simulink model "ColdGas_GNC_Model"  (R2024a)
settings: Solver=VariableStepAuto  StartTime=0.0  StopTime=tFinal  RelTol=1e-3
values from neighbouring files (symbols this model uses):
  Aero_Forces_On = 1    [run_Lander_GNC_Sim.m]
  Cd = 1.2    [Load_Aero_Data.m]
  CE_Direction = [0 0 -1]    [Load_VehicleParams.m]
  CE_ISP = 40    [Load_VehicleParams.m]
  CE_Location = [0 0 0]    [Load_VehicleParams.m]
  CE_tau = 0.100    (= 0.1)    [Load_VehicleParams.m]
  CE_tDelay = 0.030    (= 0.03)    [Load_VehicleParams.m]
  CE_Thrust = 132    [Load_VehicleParams.m]
  Cm_Lookup = [Phi'  Cm]    [Load_Aero_Data.m]
  Fan_den = [1  70.7  2500]    [Load_VehicleParams.m]
  Fan_num = 2500    [Load_VehicleParams.m]
  fan_thrust_Poly = [0.0009987  -0.04316  4.44]    [Load_VehicleParams.m]
  FlightPlan_Lateral = [0 1 5 9 13 17 20 30 30.1 30.2 2 2 ... (40 elements, 10x4)]    [Lateral_Flight_Schedule_10m.mat]    (also in Lateral_Flight_Schedule_14.mat = [0 1 11 12 13 22 29.4 29.6 29.8 30 2 2 ... (40 elements, 10x; Lateral_Flight_Schedule_15m.mat = [0 1 8.5 9 13 17 20 30 30.1 30.2 2 2 ... (40 elements, 10x4); Lateral_Flight_Schedule_2.mat = [0 3 4 6 13 17 20 30 30.1 30.2 2 2 ... (40 elements, 10x4)]; Lateral_Flight_Schedule_22.mat = [0 3 3.2 3.5 15 20 30 30.1 30.2 30.3 2 2 ... (40 elements, 1)
  FlightPlan_Vertical = [0 3 3.2 13 30 30.1 30.2 30.3 30.4 30.5 1 1 ... (30 elements, 10x3)]    [Vertical_Flight_Schedule_10m.mat]    (also in Vertical_Flight_Schedule_14.mat = [0 3 3.01 17 29 29.2 29.4 29.6 29.8 30 1 1 ... (30 elements,; Vertical_Flight_Schedule_3_15_20.mat = [0 3 3.01 15 20 29.2 29.4 29.6 29.8 30 1 1 ... (30 elements,; Vertical_Flight_Schedule_3ms.mat = [0 3 3.2 16 30 30.1 30.2 30.3 30.4 30.5 1 1 ... (30 elements)
  g = 9.807    [Load_VehicleParams.m]
  gustDuration = 9    [Load_Aero_Data.m]
  gustFactor = 1.0    (= 1)    [Load_Aero_Data.m]
  hFinal = 0.28    [run_Lander_GNC_Sim.m]
  I = [ 12  0  0 ... (first row only)    [Load_VehicleParams.m]
  LandNowFlag = false    [run_Lander_GNC_Sim.m]
  Lref = Lref_ft*0.3048    (= 0.6096)    [Load_Aero_Data.m]
  massInitial = mDry + mN2_usable + mN2_unusable    (= 47.6)    [Load_VehicleParams.m]
  Psi_Angle_deg = 5    [Load_Aero_Data.m]
  rFans = [ 0.6605    -0.6605    -0.1146 ... (first row only)    [Load_VehicleParams.m]
  rho_air = 1.2    [Load_Aero_Data.m]
  Sref = Sref_ft2*0.3048^2    (= 0.37161216)    [Load_Aero_Data.m]
  switchLines = [-3.15 -2.06213203436 1.93786796564 3.15 -3.15 -1.93786796564 2 3.15 1.89 1.89 -2.11 -2.11 ... (16 elements, 8x2)]    [PhasePlaneData.mat]
  T = 0.02    [run_Lander_GNC_Sim.m]
  t_Liftoff_Achieved = 1    [Load_VehicleParams.m]
  tau_AlgLoop = 0.01    [Load_VehicleParams.m]
  tGust_End = tGust_Start + gustDuration    (= 18)    [Load_Aero_Data.m]
  tGust_Start = 9    [Load_Aero_Data.m]
  uvFans = [ -0.1830    0.1830    -0.9659 ... (first row only)    [Load_VehicleParams.m]
  wind_angle = 0*pi/180    (= 0)    [Load_Aero_Data.m]
  windSpeed = windSpeed_knots*knots2m_per_s    [Load_Aero_Data.m]
  x0 = 0    [Load_InitialConditions.m]
  z0 = -0.3    [Load_InitialConditions.m]
undefined symbols (not defined in the file or in its folder): baseaero
libraries: matrix_library x5
settings Model: Creator=mhannan  LastModifiedBy=samue
settings SolverCC: AlgebraicLoopSolver=TrustRegion
settings OptimizationCC: DefaultParameterBehavior=Inlined  EnhancedBackFolding=on  PassReuseOutputArgsAs=Individual arguments  ZeroExternalMemoryAtStartup=off  ZeroInternalMemoryAtStartup=off  OptimizeBlockOrder=speed  DifferentSizesBufferReuse=on  EfficientTunableParamExpr=on
settings DebuggingCC: ParameterTunabilityLossMsg=error  UnconnectedInputMsg=warning  UnconnectedOutputMsg=warning  UnconnectedLineMsg=warning  ArithmeticOperatorsInVariantConditions=warning
settings ModelReferenceCC: EnableRefExpFcnMdlSchedulingChecks=on
settings SFSimCC: SimUseLocalCustomCode=off  MATLABDynamicMemAlloc=off  CustomCodeUndefinedFunction=UseInterfaceOnly
settings RTWCC: Description=Embedded Coder  SystemTargetFile=ert.tlc  TemplateMakefile=ert_default_tmf  RTWUseLocalCustomCode=off  GPUComputeCapability=3.5
settings CodeAppCC: ForceParamTrailComments=on  IgnoreCustomStorageClasses=off  OperatorAnnotations=on  SimulinkDataObjDesc=on  SFDataObjDesc=on  InsertBlockDesc=on
settings ERTTargetCC: TargetLangStandard=C99 (ISO)  GenerateSampleERTMain=on  InlinedParameterPlacement=NonHierarchical  ERTCustomFileTemplate=example_file_process.tlc

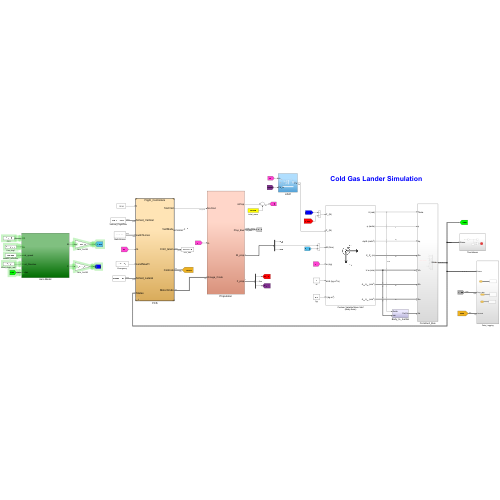
[thumbnail: Simulink's stored preview of the top-level diagram]
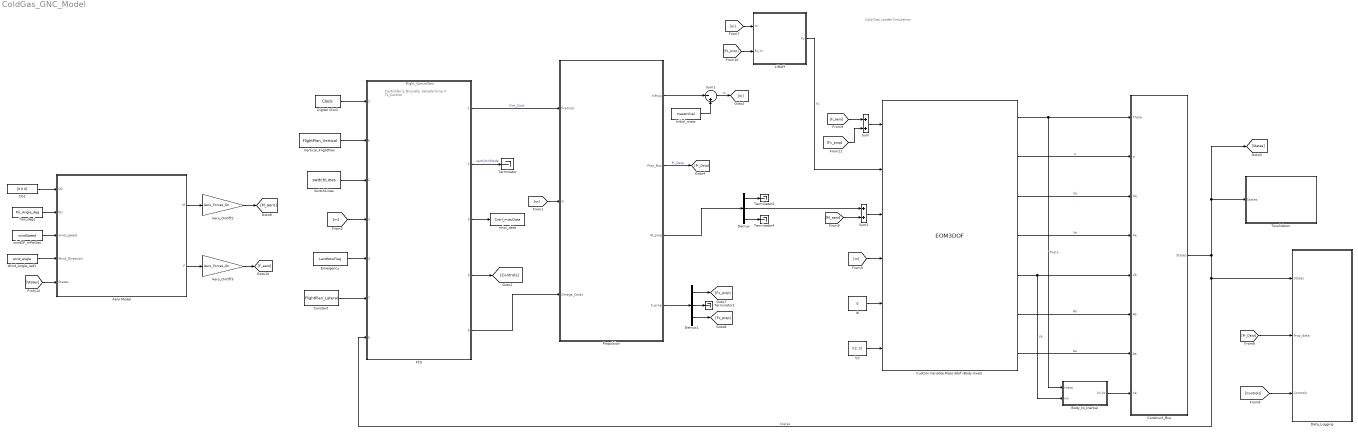
== system ColdGas_GNC_Model ==
  note: Cold Gas Lander Simulation
  note: Controller is Discrete.
      | Sample time = Ts_Control
  Aero Model : Subsystem
  Aero_OnOff2 : Gain  Gain=Aero_Forces_On
  Aero_OnOff3 : Gain  Gain=Aero_Forces_On
  Body_to_Inertial : Subsystem
  CG1 : Constant  Value=[0 0 0]
  Constant : Constant  Value=FlightPlan_Lateral
  Construct_Bus : Subsystem
  Custom Variable Mass 3dof (Body Axes) : EOM3DOF  mtype=Custom Variable  v_ini=0  theta_ini=theta0  q_ini=q0  pos_ini=[x0 z0]  abi_flag=on
  Data_Logging : Subsystem
  Demux : Demux  Outputs=3
  Demux1 : Demux  Outputs=3
  Digital Clock : DigitalClock  SampleTime=T
  Emergency : Constant  Value=LandNowFlag
  FCS : ModelReference  ModelNameDialog=Flight_Controllers.slx  SimulationMode=Normal  ModelReferenceVersion=15.21
      settings: PortSchema="{\"entries\":[{\"content\":{\"sides\":[{\"content\":{\"connectorIds\":[\"In1\",\"In6\",\"In2\",\"In3\",\"In4\",\"In7\",\"In5\"]},\"type\":\"ConnectorPlacement.EquallySpacedRectSide\",\"uuid\":\"b686e1e6-a775-4930-811b-8b7460f554d3\"},{\"content\":{\"connectorIds\":[\"Out1\",\"Out2\",\"Out3\",\"Out4\",\"Out5\"],\"side\":\"RIGHT\"},\"type\":\"ConnectorPlacement.EquallySpacedRectSide\",\"uuid\":\"9680ded8-de97-49e1-a3b4-93b1848a5220\"},{\"content\":{\"side\":\"TOP\"},\"type\":\"ConnectorPlacement.EquallySpacedRectSide\",\"uuid\":\"2545f4a3-650e-4481-9657-9ca4b463edd2\"}]},\"type\":\"ConnectorPlacement.EquallySpacedConnector\",\"uuid\":\"c05ec9f5-eee6-46c9-961b-ae1f1f81cdab\"}],\"packageUris\":[\"http://schema.mathworks.com/mf0/Connector/R2020b\"],\"version\":\"1.0\"}"
  Initial_mass : Constant  Value=massInitial
  Iyy : Constant  Value=I(2, 2)
  Liftoff : Subsystem
  Propulsion : Subsystem
  Sum : Sum
  Sum1 : Sum  Inputs=|-+
  Sum2 : Sum
  SwitchLines : Constant  Value=switchLines
  Terminator{,1..2,4} (4 alike) : Terminator
  Touchdown : Subsystem
  Vertical_FlightPlan : Constant  Value=FlightPlan_Vertical
  Wind_Angle_rad1 : Constant  Value=wind_angle
  Yaw_deg1 : Constant  Value=Psi_Angle_deg
  dI : Constant  Value=0
  misc_data : ToWorkspace  VariableName=Cntrl_miscData  SampleTime=-1
  windSP_mPerSec : Constant  Value=windSpeed
  wires:
  Sum1/1 -> [m]  "m"
  Propulsion/1(mProp) -> Sum1/1
  Initial_mass/1 -> Sum1/2
  Digital Clock/1 -> FCS/1
  FCS/1 -> Propulsion/1(fireCmd)  "Fire_Cmd"
  FCS/3 -> misc_data/1
  FCS/2 -> Terminator/1  "vertCntrlMode"
  dI/1 -> Custom Variable Mass 3dof (Body Axes)/5
  Iyy/1 -> Custom Variable Mass 3dof (Body Axes)/6
  Custom Variable Mass 3dof (Body Axes)/1 -> Body_to_Inertial/1(theta), Construct_Bus/1(Theta)  "Theta"
  Custom Variable Mass 3dof (Body Axes)/2 -> Construct_Bus/2(q)  "q"
  Custom Variable Mass 3dof (Body Axes)/3 -> Construct_Bus/3(dq)  "dq"
  Custom Variable Mass 3dof (Body Axes)/4 -> Construct_Bus/4(Xe)  "Xe"
  Custom Variable Mass 3dof (Body Axes)/5 -> Construct_Bus/5(Vb), Body_to_Inertial/2(uw)  "Vb"
  Custom Variable Mass 3dof (Body Axes)/6 -> Construct_Bus/6(Ab)  "Ab"
  Custom Variable Mass 3dof (Body Axes)/7 -> Construct_Bus/7(Ae)  "Ae"
  Construct_Bus/1(States) -> [States], Touchdown/1(States), FCS/5, Data_Logging/1(States)  "States"
  [m] -> Custom Variable Mass 3dof (Body Axes)/4
  Propulsion/2(Prop_Bus) -> [Pr_Data]  "Pr_Data"
  [Pr_Data] -> Data_Logging/2(Prop_data)
  [m] -> Liftoff/1(m)
  Liftoff/1(Fz) -> Custom Variable Mass 3dof (Body Axes)/2  "Fz"
  FCS/4 -> [Controls]
  [m] -> Propulsion/2(m)
  Propulsion/3(M_prop) -> Demux/1
  [Controls] -> Data_Logging/3(Controls)
  SwitchLines/1 -> FCS/2
  FCS/5 -> Propulsion/3(Omega_Cmds)
  Demux/1 -> Terminator2/1
  Demux/3 -> Terminator4/1
  [m] -> FCS/3
  Emergency/1 -> FCS/4
  Vertical_FlightPlan/1 -> FCS/6
  Constant/1 -> FCS/7
  [F_aero] -> Sum/1
  Sum2/1 -> Custom Variable Mass 3dof (Body Axes)/3
  Demux/2 -> Sum2/1
  [M_aero] -> Sum2/2
  Sum/1 -> Custom Variable Mass 3dof (Body Axes)/1
  Propulsion/4(F_prop) -> Demux1/1
  Demux1/1 -> [Fx_prop]
  Demux1/2 -> Terminator1/1
  Demux1/3 -> [Fz_prop]
  [Fz_prop] -> Liftoff/2(Fz_In)
  [Fx_prop] -> Sum/2
  Body_to_Inertial/1(Vx,Vz) -> Construct_Bus/8(Ve)
  [States] -> Aero Model/5(States)
  Wind_Angle_rad1/1 -> Aero Model/4(Wind_Direction)
  windSP_mPerSec/1 -> Aero Model/3(wind_speed)
  Yaw_deg1/1 -> Aero Model/2(Psi)
  CG1/1 -> Aero Model/1(CG)
  Aero Model/1(M) -> Aero_OnOff2/1
  Aero_OnOff2/1 -> [M_aero]
  Aero Model/2(F) -> Aero_OnOff3/1
  Aero_OnOff3/1 -> [F_aero]

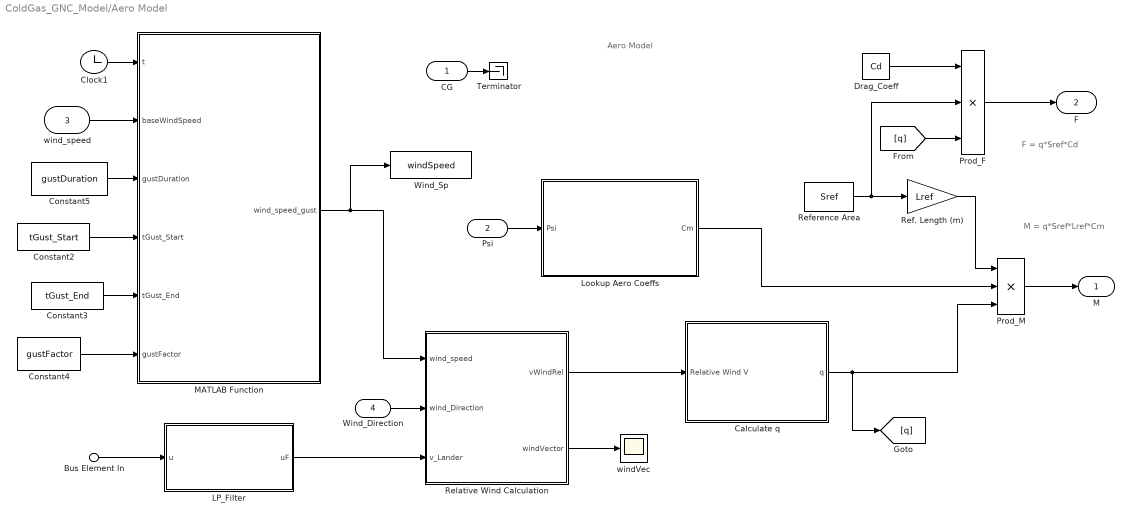
== system ColdGas_GNC_Model/Aero Model ==
  note: Aero Model
  note: F = q*Sref*Cd
  note: M = q*Sref*Lref*Cm
  CG : Inport
  Psi : Inport  Port=2
  wind_speed : Inport  Port=3
  Wind_Direction : Inport  Port=4
  Bus Element In : Inport  Port=5  PortName=States  Element=VxE
  Calculate q : Subsystem
  Clock1 : Clock
  Constant2 : Constant  Value=tGust_Start
  Constant3 : Constant  Value=tGust_End
  Constant4 : Constant  Value=gustFactor
  Constant5 : Constant  Value=gustDuration
  Drag_Coeff : Constant  Value=Cd
  LP_Filter : Subsystem
  Lookup Aero Coeffs : Subsystem
  MATLAB Function : MATLAB Function  TreatAsAtomicUnit=on
  Prod_F : Product  Inputs=3  RndMeth=Zero
  Prod_M : Product  Inputs=3  RndMeth=Zero
  Ref. Length (m) : Gain  Gain=Lref
  Reference Area : Constant  Value=Sref
  Relative Wind Calculation : Subsystem
  Terminator : Terminator
  Wind_Sp : ToWorkspace  VariableName=windSpeed  SaveFormat=Timeseries  SampleTime=-1
  windVec : Scope
  M : Outport
  F : Outport  Port=2
  wires:
  Relative Wind Calculation/1(vWindRel) -> Calculate q/1(Relative Wind V)
  Reference Area/1 -> Prod_F/2, Ref. Length (m)/1
  Calculate q/1(q) -> [q], Prod_M/3
  Ref. Length (m)/1 -> Prod_M/1
  [q] -> Prod_F/3
  Psi/1 -> Lookup Aero Coeffs/1(Psi)
  Wind_Direction/1 -> Relative Wind Calculation/2(wind_Direction)
  CG/1 -> Terminator/1
  wind_speed/1 -> MATLAB Function/2(baseWindSpeed)
  Drag_Coeff/1 -> Prod_F/1
  Lookup Aero Coeffs/1(Cm) -> Prod_M/2
  Prod_M/1 -> M/1
  Prod_F/1 -> F/1
  Bus Element In/1 -> LP_Filter/1(u)
  LP_Filter/1(uF) -> Relative Wind Calculation/3(v_Lander)
  Clock1/1 -> MATLAB Function/1(t)
  MATLAB Function/1(wind_speed_gust) -> Wind_Sp/1, Relative Wind Calculation/1(wind_speed)
  Constant2/1 -> MATLAB Function/4(tGust_Start)
  Constant3/1 -> MATLAB Function/5(tGust_End)
  Constant4/1 -> MATLAB Function/6(gustFactor)
  Constant5/1 -> MATLAB Function/3(gustDuration)
  Relative Wind Calculation/2(windVector) -> windVec/1

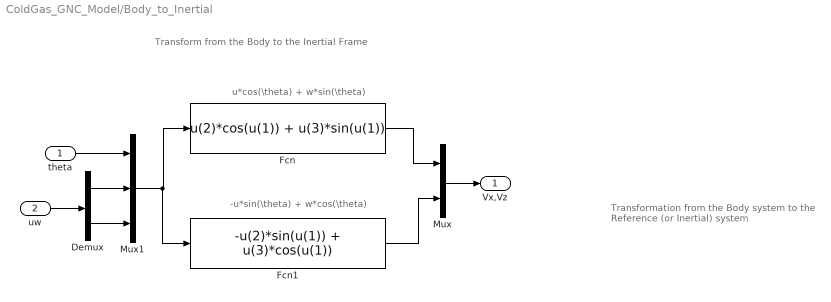
== system ColdGas_GNC_Model/Body_to_Inertial ==
  note: Transformation from the Body system to the Reference (or Inertial) system
  note: Transform from the Body to the Inertial Frame
  note: u*cos(\theta) + w*sin(\theta)
  note: -u*sin(\theta) + w*cos(\theta)
  theta : Inport
  uw : Inport  Port=2
  Demux : Demux  Outputs=2
  Fcn : Fcn  Expr=u(2)*cos(u(1)) + u(3)*sin(u(1))
  Fcn1 : Fcn  Expr=-u(2)*sin(u(1)) + u(3)*cos(u(1))
  Mux : Mux  Inputs=2
  Mux1 : Mux  Inputs=3
  Vx,Vz : Outport  VectorParamsAs1DForOutWhenUnconnected=off
  wires:
  uw/1 -> Demux/1
  theta/1 -> Mux1/1
  Demux/1 -> Mux1/2
  Demux/2 -> Mux1/3
  Fcn/1 -> Mux/1
  Fcn1/1 -> Mux/2
  Mux/1 -> Vx,Vz/1
  Mux1/1 -> Fcn1/1, Fcn/1

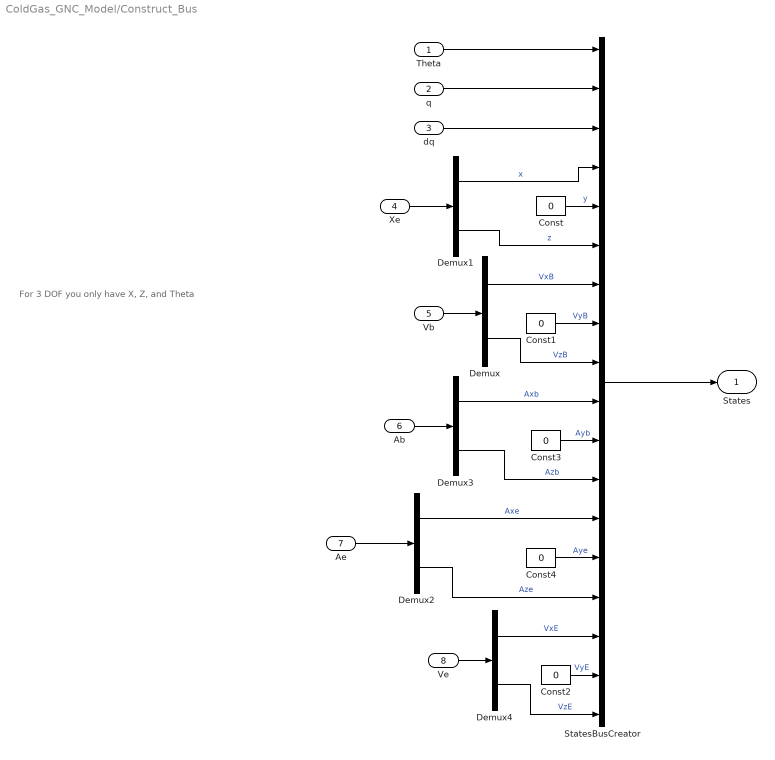
== system ColdGas_GNC_Model/Construct_Bus ==
  note: For 3 DOF you only have X, Z, and Theta
  Theta : Inport
  q : Inport  Port=2
  dq : Inport  Port=3
  Xe : Inport  Port=4
  Vb : Inport  Port=5
  Ab : Inport  Port=6
  Ae : Inport  Port=7
  Ve : Inport  Port=8
  Const{,1..4} (5 alike) : Constant  Value=0
  Demux{,1..4} (5 alike) : Demux  Outputs=2
  StatesBusCreator : BusCreator  Inputs=18  OutDataTypeStr=Bus: States  NonVirtualBus=on
  States : Outport
  wires:
  dq/1 -> StatesBusCreator/3
  StatesBusCreator/1 -> States/1
  Theta/1 -> StatesBusCreator/1
  q/1 -> StatesBusCreator/2
  Demux/1 -> StatesBusCreator/7  "VxB"
  Demux1/1 -> StatesBusCreator/4  "x"
  Xe/1 -> Demux1/1
  Vb/1 -> Demux/1
  Demux3/1 -> StatesBusCreator/10  "Axb"
  Ab/1 -> Demux3/1
  Ae/1 -> Demux2/1
  Demux2/1 -> StatesBusCreator/13  "Axe"
  Const/1 -> StatesBusCreator/5  "y"
  Demux1/2 -> StatesBusCreator/6  "z"
  Const1/1 -> StatesBusCreator/8  "VyB"
  Demux/2 -> StatesBusCreator/9  "VzB"
  Const3/1 -> StatesBusCreator/11  "Ayb"
  Demux3/2 -> StatesBusCreator/12  "Azb"
  Const4/1 -> StatesBusCreator/14  "Aye"
  Demux2/2 -> StatesBusCreator/15  "Aze"
  Demux4/1 -> StatesBusCreator/16  "VxE"
  Demux4/2 -> StatesBusCreator/18  "VzE"
  Const2/1 -> StatesBusCreator/17  "VyE"
  Ve/1 -> Demux4/1

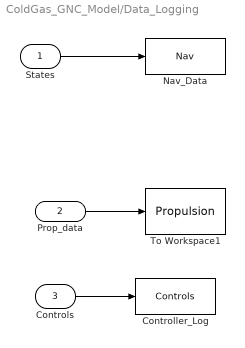
== system ColdGas_GNC_Model/Data_Logging ==
  States : Inport
  Prop_data : Inport  Port=2
  Controls : Inport  Port=3
  Controller_Log : ToWorkspace  VariableName=Controls  SaveFormat=Timeseries  SampleTime=-1
  Nav_Data : ToWorkspace  VariableName=Nav  SaveFormat=Timeseries  SampleTime=-1
  To Workspace1 : ToWorkspace  VariableName=Propulsion  SaveFormat=Timeseries  SampleTime=-1
  wires:
  Controls/1 -> Controller_Log/1
  Prop_data/1 -> To Workspace1/1
  States/1 -> Nav_Data/1

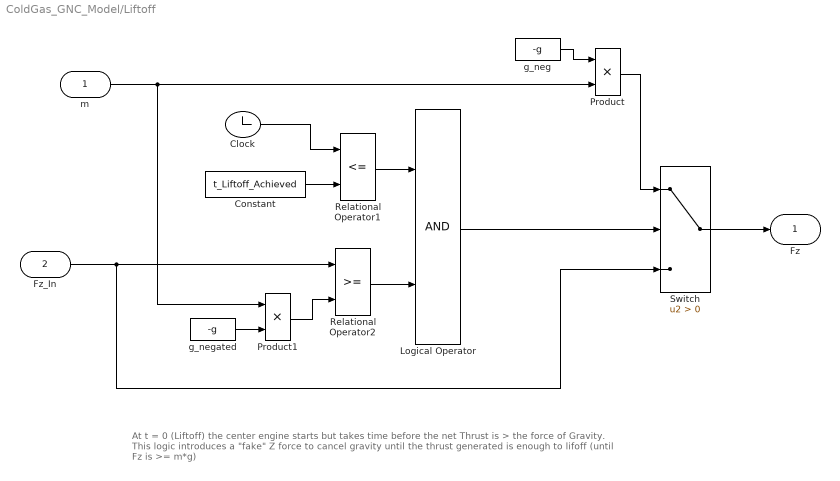
== system ColdGas_GNC_Model/Liftoff ==
  note: At t = 0 (Liftoff) the center engine starts but takes time before the net Thrust is > the force of Gravity. This logic introduces a "fake" Z force to cancel gravity until the thrust generated is enough to lifoff (until Fz is >= m*g)
  m : Inport
  Fz_In : Inport  Port=2
  Clock : Clock
  Constant : Constant  Value=t_Liftoff_Achieved
  Logical Operator : Logic  AllPortsSameDT=off  OutDataTypeStr=boolean
  Product : Product
  Product1 : Product
  Relational Operator1 : RelationalOperator  Operator=<=  OutDataTypeStr=boolean  RndMeth=Simplest  InputSameDT=off
  Relational Operator2 : RelationalOperator  OutDataTypeStr=boolean  RndMeth=Simplest  InputSameDT=off
  Switch : Switch  Criteria=u2 > Threshold  SaturateOnIntegerOverflow=off  InputSameDT=off
  g_neg : Constant  Value=-g
  g_negated : Constant  Value=-g
  Fz : Outport
  wires:
  Clock/1 -> Relational Operator1/1
  Constant/1 -> Relational Operator1/2
  Relational Operator1/1 -> Logical Operator/1
  Fz_In/1 -> Relational Operator2/1, Switch/3
  Logical Operator/1 -> Switch/2
  Switch/1 -> Fz/1
  Relational Operator2/1 -> Logical Operator/2
  g_neg/1 -> Product/1
  Product/1 -> Switch/1
  g_negated/1 -> Product1/2
  Product1/1 -> Relational Operator2/2
  m/1 -> Product1/1, Product/2

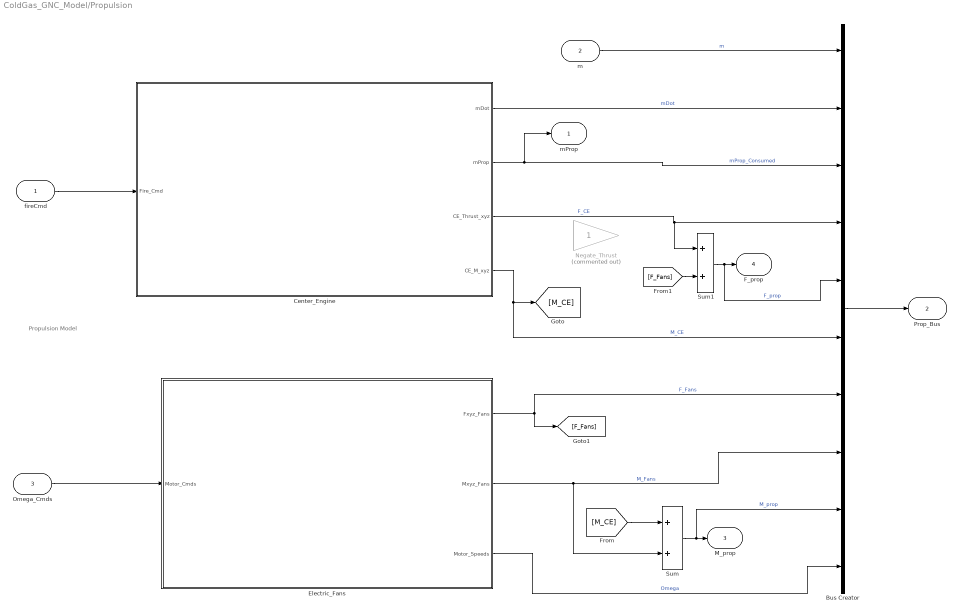
== system ColdGas_GNC_Model/Propulsion ==
  note: Propulsion Model
  fireCmd : Inport
  m : Inport  Port=2
  Omega_Cmds : Inport  Port=3
  Bus Creator : BusCreator  Inputs=10
  Center_Engine : Subsystem
  Electric_Fans : Subsystem
  Negate_Thrust : Gain  Commented=on
  Sum : Sum
  Sum1 : Sum
  mProp : Outport
  Prop_Bus : Outport  Port=2
  M_prop : Outport  Port=3
  F_prop : Outport  Port=4
  wires:
  Bus Creator/1 -> Prop_Bus/1
  fireCmd/1 -> Center_Engine/1(Fire_Cmd)
  Center_Engine/1(mDot) -> Bus Creator/2  "mDot"
  Center_Engine/2(mProp) -> Bus Creator/3, mProp/1  "mProp_Consumed"
  Center_Engine/3(CE_Thrust_xyz) -> Sum1/1, Bus Creator/4  "F_CE"
  Electric_Fans/3(Motor_Speeds) -> Bus Creator/10  "Omega"
  Electric_Fans/1(Fxyz_Fans) -> [F_Fans], Bus Creator/7  "F_Fans"
  Omega_Cmds/1 -> Electric_Fans/1(Motor_Cmds)
  m/1 -> Bus Creator/1  "m"
  Center_Engine/4(CE_M_xyz) -> [M_CE], Bus Creator/6  "M_CE"
  Electric_Fans/2(Mxyz_Fans) -> Bus Creator/8, Sum/2  "M_Fans"
  [M_CE] -> Sum/1
  Sum/1 -> Bus Creator/9, M_prop/1  "M_prop"
  Sum1/1 -> Bus Creator/5, F_prop/1  "F_prop"
  [F_Fans] -> Sum1/2

== system ColdGas_GNC_Model/Touchdown ==
  Bus Element In : Inport  PortName=States  Element=z
  End : Stop
  Gain : Gain  Gain=-1
  Pos : ToWorkspace  VariableName=h  SaveFormat=Timeseries  SampleTime=-1
  Relational Operator : RelationalOperator  Operator=<=  OutDataTypeStr=boolean  RndMeth=Simplest  InputSameDT=off
  Stop_Altitude : Constant  Value=hFinal
  wires:
  Stop_Altitude/1 -> Relational Operator/2
  Relational Operator/1 -> End/1
  Bus Element In/1 -> Gain/1
  Gain/1 -> Relational Operator/1, Pos/1

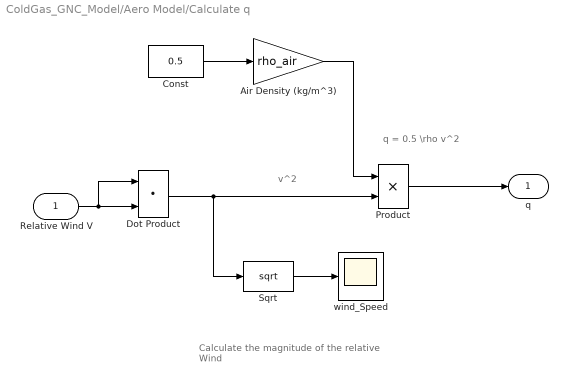
== system ColdGas_GNC_Model/Aero Model/Calculate q ==
  note: Calculate the magnitude
      | of the relative Wind
  note: q = 0.5 \rho v^2
  note: v^2
  Relative Wind V : Inport
  Air Density (kg/m^3) : Gain  Gain=rho_air
  Const : Constant  Value=0.5
  Dot Product : DotProduct  OutDataTypeStr=Inherit: Inherit via internal rule
  Product : Product  RndMeth=Zero
  Sqrt : Sqrt
  wind_Speed : Scope
  q : Outport
  wires:
  Relative Wind V/1 -> Dot Product/1, Dot Product/2
  Dot Product/1 -> Product/2, Sqrt/1
  Const/1 -> Air Density (kg/m^3)/1
  Air Density (kg/m^3)/1 -> Product/1
  Product/1 -> q/1
  Sqrt/1 -> wind_Speed/1

== system ColdGas_GNC_Model/Aero Model/LP_Filter ==
  u : Inport
  Int_LP : Integrator
  Sum3 : Sum  Inputs=|+-
  one_over_tau : Gain  Gain=1/tau_AlgLoop
  uF : Outport
  wires:
  Sum3/1 -> one_over_tau/1
  u/1 -> Sum3/1
  Int_LP/1 -> uF/1, Sum3/2
  one_over_tau/1 -> Int_LP/1

== system ColdGas_GNC_Model/Aero Model/Lookup Aero Coeffs ==
  note: Lookup the coefficients in the Aero Database.
  Psi : Inport
  Cm Lookup Table (n-D) : Lookup_n-D  NumberOfTableDimensions=1  BreakpointsForDimension1=Cm_Lookup(:,1)  BreakpointsForDimension2=baseaero.Cm.V.Theta  Table=Cm_Lookup(:,2)
  Display : Display
  Cm : Outport
  wires:
  Psi/1 -> Cm Lookup Table (n-D)/1
  Cm Lookup Table (n-D)/1 -> Display/1, Cm/1  "Cm"

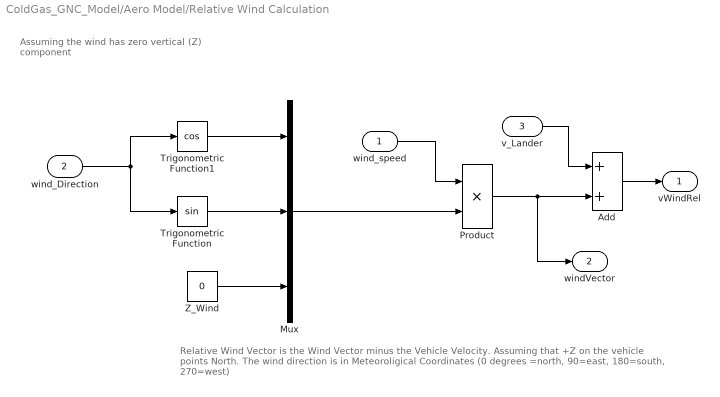
== system ColdGas_GNC_Model/Aero Model/Relative Wind Calculation ==
  note: Relative Wind Vector is the Wind Vector minus the Vehicle Velocity.
      | Assuming that +Z on the vehicle points North.
      | The wind direction is in Meteoroligical Coordinates
      |                    (0 degrees =north, 90=east, 180=south, 270=west)
  note: Assuming the wind has
      | zero vertical (Z) component
  wind_speed : Inport
  wind_Direction : Inport  Port=2
  v_Lander : Inport  Port=3
  Add : Sum
  Mux : Mux  Inputs=3
  Product : Product  RndMeth=Zero
  Trigonometric Function : Trigonometry
  Trigonometric Function1 : Trigonometry  Operator=cos
  Z_Wind : Constant  Value=0
  vWindRel : Outport
  windVector : Outport  Port=2
  wires:
  Mux/1 -> Product/2
  Product/1 -> windVector/1, Add/2
  Add/1 -> vWindRel/1
  wind_Direction/1 -> Trigonometric Function/1, Trigonometric Function1/1
  Trigonometric Function1/1 -> Mux/1
  Trigonometric Function/1 -> Mux/2
  Z_Wind/1 -> Mux/3
  wind_speed/1 -> Product/1
  v_Lander/1 -> Add/1

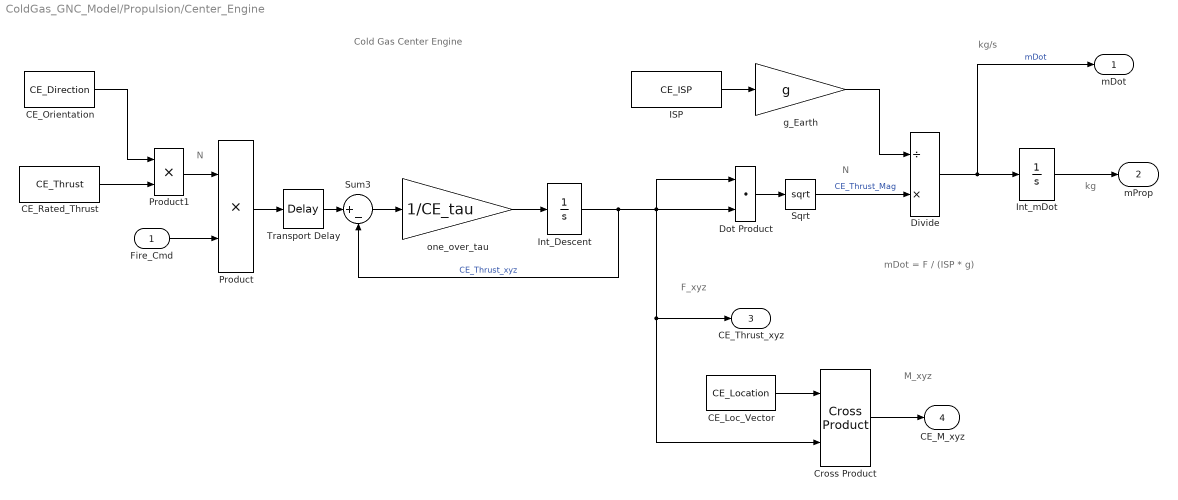
== system ColdGas_GNC_Model/Propulsion/Center_Engine ==
  note: N
  note: Cold Gas Center Engine
  note: mDot = F / (ISP * g)
  note: N
  note: kg
  note: kg/s
  note: F_xyz
  note: M_xyz
  Fire_Cmd : Inport
  CE_Loc_Vector : Constant  Value=CE_Location
  CE_Orientation : Constant  Value=CE_Direction
  CE_Rated_Thrust : Constant  Value=CE_Thrust
  Cross Product : matrix_library/Cross Product
  Divide : Product  Inputs=/*
  Dot Product : DotProduct  OutDataTypeStr=Inherit: Inherit via internal rule
  ISP : Constant  Value=CE_ISP
  Int_Descent : Integrator
  Int_mDot : Integrator
  Product : Product
  Product1 : Product
  Sqrt : Sqrt
  Sum3 : Sum  Inputs=|+-
  Transport Delay : TransportDelay  DelayTime=CE_tDelay
  g_Earth : Gain  Gain=g
  one_over_tau : Gain  Gain=1/CE_tau
  mDot : Outport
  mProp : Outport  Port=2
  CE_Thrust_xyz : Outport  Port=3
  CE_M_xyz : Outport  Port=4
  wires:
  g_Earth/1 -> Divide/1
  Int_Descent/1 -> Sum3/2, Dot Product/2, Dot Product/1, CE_Thrust_xyz/1, Cross Product/2  "CE_Thrust_xyz"
  ISP/1 -> g_Earth/1
  Product/1 -> Transport Delay/1
  CE_Rated_Thrust/1 -> Product1/2
  Int_mDot/1 -> mProp/1
  Transport Delay/1 -> Sum3/1
  Sum3/1 -> one_over_tau/1
  Divide/1 -> mDot/1, Int_mDot/1  "mDot"
  one_over_tau/1 -> Int_Descent/1
  Fire_Cmd/1 -> Product/2
  Product1/1 -> Product/1
  CE_Orientation/1 -> Product1/1
  Dot Product/1 -> Sqrt/1
  Sqrt/1 -> Divide/2  "CE_Thrust_Mag"
  CE_Loc_Vector/1 -> Cross Product/1
  Cross Product/1 -> CE_M_xyz/1

== system ColdGas_GNC_Model/Propulsion/Electric_Fans ==
  note: Calculate the Forces and Moments from the 4 Electric Fans
  note: kg
  Motor_Cmds : Inport
  Determine_Motor_Speeds : Subsystem
  Moments : Subsystem
  Fxyz_Fans : Outport
  Mxyz_Fans : Outport  Port=2
  Motor_Speeds : Outport  Port=3
  wires:
  Determine_Motor_Speeds/2(Thrust_motors) -> Moments/1(Thrust_Motors)
  Moments/1(M_xyz) -> Mxyz_Fans/1
  Moments/2(F_xyz) -> Fxyz_Fans/1
  Determine_Motor_Speeds/1(Omega_Motors) -> Motor_Speeds/1
  Motor_Cmds/1 -> Determine_Motor_Speeds/1(MotorCmd_Bus)

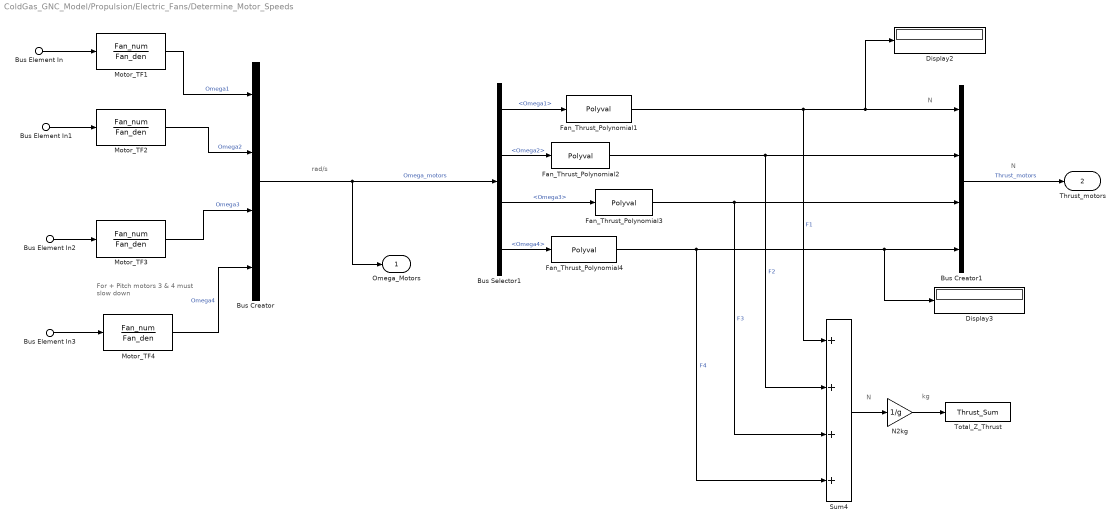
== system ColdGas_GNC_Model/Propulsion/Electric_Fans/Determine_Motor_Speeds ==
  note: kg
  note: N
  note: For + Pitch motors
      | 3 & 4 must slow down
  note: N
  note: rad/s
  note: N
  Bus Element In : Inport  PortName=MotorCmd_Bus  Element=M1
  Bus Element In1 : Inport  PortName=MotorCmd_Bus  Element=M2
  Bus Element In2 : Inport  PortName=MotorCmd_Bus  Element=M3
  Bus Element In3 : Inport  PortName=MotorCmd_Bus  Element=M4
  Bus Creator : BusCreator  Inputs=4
  Bus Creator1 : BusCreator  Inputs=4
  Bus Selector1 : BusSelector  OutputSignals=Omega1,Omega2,Omega3,Omega4
  Display2 : Display
  Display3 : Display
  Fan_Thrust_Polynomial{1..4} (4 alike) : Polyval  Coefs=fan_thrust_Poly
  Motor_TF{1..4} (4 alike) : TransferFcn  Numerator=Fan_num  Denominator=Fan_den
  N2kg : Gain  Gain=1/g
  Sum4 : Sum  Inputs=++++
  Total_Z_Thrust : ToWorkspace  VariableName=Thrust_Sum  SaveFormat=Timeseries  SampleTime=-1
  Omega_Motors : Outport
  Thrust_motors : Outport  Port=2
  wires:
  Bus Selector1/2 -> Fan_Thrust_Polynomial2/1  "<Omega2>"
  Bus Creator/1 -> Omega_Motors/1, Bus Selector1/1  "Omega_motors"
  Fan_Thrust_Polynomial1/1 -> Display2/1, Bus Creator1/1, Sum4/1  "F1"
  Bus Selector1/4 -> Fan_Thrust_Polynomial4/1  "<Omega4>"
  Fan_Thrust_Polynomial3/1 -> Bus Creator1/3, Sum4/3  "F3"
  Bus Selector1/3 -> Fan_Thrust_Polynomial3/1  "<Omega3>"
  Bus Selector1/1 -> Fan_Thrust_Polynomial1/1  "<Omega1>"
  Sum4/1 -> N2kg/1
  Fan_Thrust_Polynomial2/1 -> Sum4/2, Bus Creator1/2  "F2"
  Fan_Thrust_Polynomial4/1 -> Display3/1, Bus Creator1/4, Sum4/4  "F4"
  N2kg/1 -> Total_Z_Thrust/1
  Bus Creator1/1 -> Thrust_motors/1  "Thrust_motors"
  Motor_TF1/1 -> Bus Creator/1  "Omega1"
  Motor_TF2/1 -> Bus Creator/2  "Omega2"
  Motor_TF3/1 -> Bus Creator/3  "Omega3"
  Motor_TF4/1 -> Bus Creator/4  "Omega4"
  Bus Element In/1 -> Motor_TF1/1
  Bus Element In1/1 -> Motor_TF2/1
  Bus Element In2/1 -> Motor_TF3/1
  Bus Element In3/1 -> Motor_TF4/1

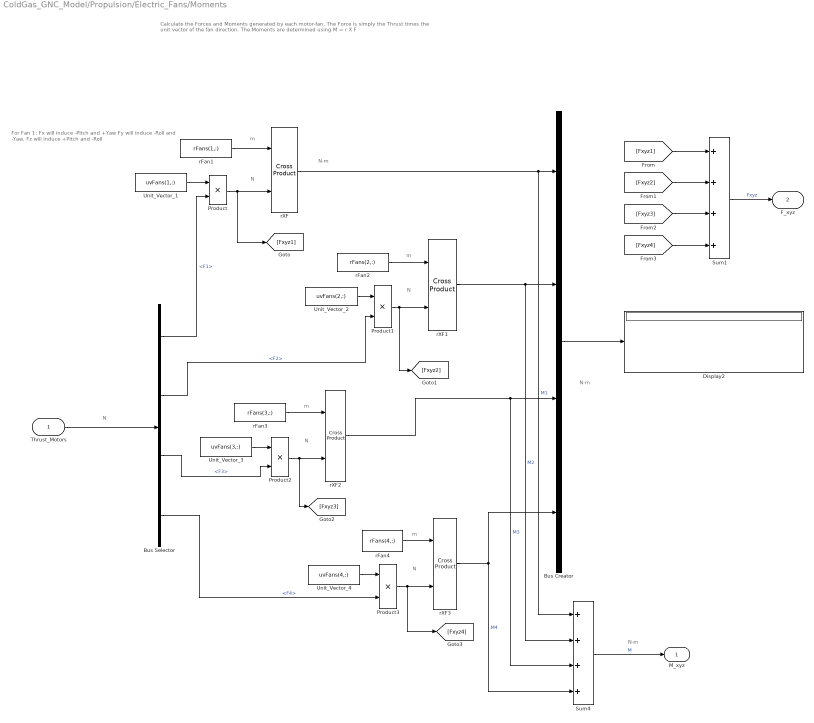
== system ColdGas_GNC_Model/Propulsion/Electric_Fans/Moments ==
  note: Calculate the Forces and Moments generated by each motor-fan.
      | The Force is simply the Thrust times the unit vector of the fan direction.
      | The Moments are determined using M = r X F
  note: N-m
  note: N
  note: m
  note: For Fan 1: Fx will induce -Pitch and +Yaw
      | Fy will induce -Roll and -Yaw.
      | Fz will induce +Pitch and -Roll
  note: m
  note: N
  note: N
  note: m
  note: N
  note: m
  note: N
  note: N-m
  note: N-m
  Thrust_Motors : Inport
  Bus Creator : BusCreator  Inputs=4
  Bus Selector : BusSelector  OutputSignals=F1,F2,F3,F4
  Display2 : Display
  Product{,1..3} (4 alike) : Product
  Sum1 : Sum  Inputs=++++
  Sum4 : Sum  Inputs=++++
  Unit_Vector_1 : Constant  Value=uvFans(1,:)
  Unit_Vector_2 : Constant  Value=uvFans(2,:)
  Unit_Vector_3 : Constant  Value=uvFans(3,:)
  Unit_Vector_4 : Constant  Value=uvFans(4,:)
  rFan1 : Constant  Value=rFans(1,:)
  rFan2 : Constant  Value=rFans(2,:)
  rFan3 : Constant  Value=rFans(3,:)
  rFan4 : Constant  Value=rFans(4,:)
  rXF{,1..3} (4 alike) : matrix_library/Cross Product
  M_xyz : Outport
  F_xyz : Outport  Port=2
  wires:
  Product/1 -> [Fxyz1], rXF/2
  Bus Selector/1 -> Product/2  "<F1>"
  rFan3/1 -> rXF2/1
  Unit_Vector_1/1 -> Product/1
  rXF1/1 -> Bus Creator/2, Sum4/2  "M2"
  rFan1/1 -> rXF/1
  Unit_Vector_3/1 -> Product2/1
  Unit_Vector_2/1 -> Product1/1
  rXF3/1 -> Bus Creator/4, Sum4/4  "M4"
  rXF2/1 -> Bus Creator/3, Sum4/3  "M3"
  Product2/1 -> [Fxyz3], rXF2/2
  rFan2/1 -> rXF1/1
  Product1/1 -> [Fxyz2], rXF1/2
  rXF/1 -> Sum4/1, Bus Creator/1  "M1"
  Bus Selector/4 -> Product3/2  "<F4>"
  Unit_Vector_4/1 -> Product3/1
  Sum4/1 -> M_xyz/1  "M"
  Bus Selector/2 -> Product1/2  "<F2>"
  Bus Selector/3 -> Product2/2  "<F3>"
  rFan4/1 -> rXF3/1
  Product3/1 -> [Fxyz4], rXF3/2
  Bus Creator/1 -> Display2/1
  Thrust_Motors/1 -> Bus Selector/1
  [Fxyz1] -> Sum1/1
  Sum1/1 -> F_xyz/1  "Fxyz"
  [Fxyz2] -> Sum1/2
  [Fxyz3] -> Sum1/3
  [Fxyz4] -> Sum1/4

== matlab function ColdGas_GNC_Model/Aero Model/MATLAB Function ==
  data: t input; wind_speed_gust output; baseWindSpeed input; gustDuration input; tGust_Start input; tGust_End input; gustFactor input
function wind_speed_gust = wind_gust(t, baseWindSpeed, gustDuration, tGust_Start, tGust_End, gustFactor)
%UNTITLED Summary of this function goes here
%   Detailed explanation goes here

if t  >=  tGust_Start   &&    t <=  tGust_End
    wind_speed_gust = baseWindSpeed*(gustFactor - 1) * ...
                                  0.5*(1 - cos(2*pi*(t - tGust_Start)/gustDuration))  +  baseWindSpeed;
else
    wind_speed_gust  =  baseWindSpeed;
end

end
